simulink model "projectme548"  (R2016a)
settings: Solver=ode45  SolverMode=SingleTasking  StartTime=0.0  StopTime=5  MaxStep=0.01  RelTol=1e-3
model workspace (MAT data in the model file):
  A = 29.46
  Cd = 0.27
  Converter_K = [105 107 109 110 111 118 120 130 140 158 600]
  Converter_K2 = [138 139 138 138 139 140 142 145 155 165 200]
  Converter_K3 = [137.465208994; 137.065019157; 135.864449646; 135.664354728; 137.565256453; 140.366585312; 145.268910814; 152.872517717; 162.9773111; 164.27792807; 166.178829795; 167.979684062; 170.080680706; 172.781962105; 175.383196045; 179.585189333; 183.587087703; 189.890077635; 197.693779455; 215.902417037; 244.515990379]
  Converter_sratio = [0 0.1 0.2 0.3 0.4 0.5 0.6 0.7 0.8 0.9 1]
  Converter_sratio3 = [0 0.1 0.2 0.3 0.4 0.5 0.6 0.7 0.8 0.81 0.82 0.83 0.84 0.85 0.86 0.87 0.88 0.89 0.9 0.92 0.94]
  Converter_tratio = [2.1 2.03 1.93 1.82 1.7 1.58 1.42 1.3 1.17 1 1]
  Converter_tratio3 = [2.232 2.075 1.975 1.846 1.72 1.564 1.409 1.254 1.096 1.08 1.061 1.043 1.028 1.012 1.002 1.002 1.001 0.998 1 1.001 1.002]
  Engine_speed = [1000 1500 2000 2500 3000 3500 4000 4500 5000 5500 6000 6500 7000]
  Engine_torque = [140 152 156 167 164 167 169 175 171 165 159 150 138]
  Engine_torque2 = [160 170 185 190 198 205 210 170 160 150 140 145 120]
  Engine_torque3 = [134.973873267 156.363175588 165.213921376 168.901732121 173.327105015 175.539791462 173.327105015 169.63929427 162.26367278 147.5124298 132.76118682 88.50745788 59.00497192]
  G = 0
  I_c1r2 = 0.02
  I_c2r3 = 0.02
  I_input = 0.02
  I_out = 0.02
  I_s1 = 0.02
  I_s3 = 0.02
  Iv = 8.97221507589
  Je = 0.3
  T_C = [0 7 11.9677 49 80.1613 93.2581 98.6774 99.129 98.6774 98.2258 98.6774 99.5806 98.6774 98.2258 97.3226 102.2903 109.9677 133.4516 134.3548]
  W = 3472
  ans = 0.94
  f = 0.018
  g = 32.2
  ia = 2.6
  r = 0.75
undefined symbols (not defined in the file): magnitude, sigbuilder_block
settings Model: PauseTimes=1  Creator=eiddie  LastModifiedBy=xiaohuil
settings DataIOCC: LimitDataPoints=on  SaveFormat=Array
settings OptimizationCC: BlockReduction=off  BooleanDataType=off
settings DebuggingCC: SaveWithParameterizedLinksMsg=none  UnderspecifiedInitializationDetection=Classic  MergeDetectMultiDrivingBlocksExec=none  SignalResolutionControl=TryResolveAllWithWarning
settings HardwareCC: ProdBitPerPointer=32  ProdLargestAtomicFloat=None  ProdIntDivRoundTo=Undefined  ProdEndianess=Unspecified  ProdWordSize=32  ProdHWDeviceType=32-bit Generic  TargetUnknown=on
settings ModelReferenceCC: PropagateSignalLabelsOutOfModel=off
settings ConfigComp: CovModelRefEnable=Off  CovSFcnEnable=off

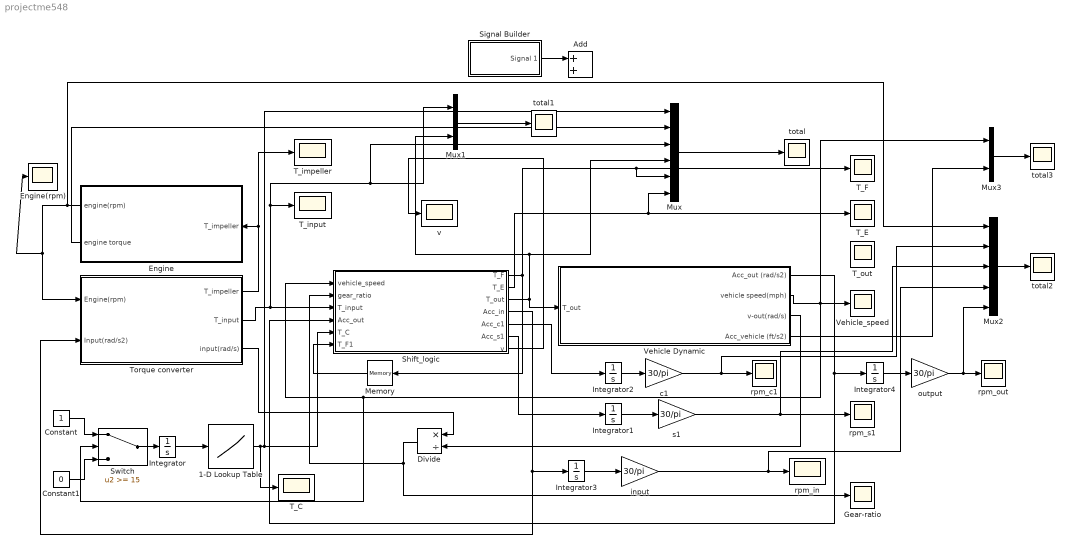
== system projectme548 ==
  1-D Lookup Table : Lookup_n-D  NumberOfTableDimensions=1  BreakpointsForDimension1=[0,0.1,0.2,0.3,0.4,0.5,0.6,0.7,0.8,0.9,1,1.1,1.2,1.3,1.4,1.5,1.6,1.7,1.8]  Table=T_C  InternalRulePriority=Speed  RndMeth=Simplest  InputSameDT=on
  Add : Sum
  Constant : Constant
  Constant1 : Constant  Value=0
  Divide : Product  Inputs=*/
  Engine : Subsystem
  Engine(rpm) : Scope
  Gear-ratio : Scope
  Integrator{,1..4} (5 alike) : Integrator
  Memory : Memory  X0=1
  Mux : Mux  Inputs=6
  Mux1 : Mux  Inputs=2
  Mux2 : Mux  Inputs=5
  Mux3 : Mux  Inputs=2
  Shift_logic : MATLAB Function  TreatAsAtomicUnit=on
      settings: MinAlgLoopOccurrences=on
  Signal Builder : Subsystem  Tag=STV Subsys  LoadFcn=sigbuilder_block('load');  StartFcn=sigbuilder_block('start');  StopFcn=sigbuilder_block('stop');  ClipboardFcn=sigbuilder_block('clipboard');  mask(Sigbuilder block){}
      mask help: Simulink:masks:SigbuilderBlock_MD
      mask init:
      | if ~strcmp(get_param(bdroot(gcbh),'SimulationStatus'),'stopped') tuvar = sigbuilder_block('maskInit'); end
      settings: CopyFcn=sigbuilder_block('copy');  DeleteFcn=sigbuilder_block('delete');  ModelCloseFcn=sigbuilder_block('modelClose');  PreSaveFcn=sigbuilder_block('preSave');  PauseFcn=sigbuilder_block('pause');  ContinueFcn=sigbuilder_block('continue');  NameChangeFcn=sigbuilder_block('namechange');  OpenFcn=sigbuilder_block('open',[437.6 199.2 550.4 400 ]);  CloseFcn=sigbuilder_block('close');
      mask Display: plot(0, 0, 100, 100,[2, 2, 32, 32, 2], [68, 8, 8, 68, 68],[32, 2], [38, 38], [32, 19, 2],[53, 60, 44], [32, 17, 17, 2],[16, 16, 31, 31]);txt = getActiveGroup(gcbh);text(2, 100, txt,'verticalAlignment', 'top');
  Switch : Switch  Threshold=15
  T_C : Scope
  T_E : Scope
  T_F : Scope
  T_impeller : Scope
  T_input : Scope
  T_out : Scope
  Torque converter : Subsystem
  Vehicle Dynamic : Subsystem
  Vehicle_speed : Scope
  c1 : Gain  Gain=30/pi
  input : Gain  Gain=30/pi
  output : Gain  Gain=30/pi
  rpm_c1 : Scope
  rpm_in : Scope
  rpm_out : Scope
  rpm_s1 : Scope
  s1 : Gain  Gain=30/pi
  total{,1..3} (4 alike) : Scope
  "v " : Scope
  wires:
  Engine/1(engine(rpm)) -> Torque converter/1(Engine(rpm)), Engine(rpm)/1, Mux2/1
  Torque converter/1(T_impeller) -> T_impeller/1, Engine/1(T_impeller)
  Torque converter/2(T_input) -> Shift_logic/3(T_input), Mux1/1, Mux/3, T_input/1
  Shift_logic/3(T_out) -> Mux1/2, Mux/4, Vehicle Dynamic/1(T_out)
  Shift_logic/2(T_E) -> Mux/6, T_E/1
  Shift_logic/6(Acc_s1) -> Integrator1/1
  Constant1/1 -> Switch/3
  Constant/1 -> Switch/1
  Switch/1 -> Integrator/1
  Integrator/1 -> 1-D Lookup Table/1
  1-D Lookup Table/1 -> Mux/1, Shift_logic/5(T_C), T_C/1
  Shift_logic/1(T_F) -> Memory/1, Mux/5, T_F/1
  Vehicle Dynamic/3(v-out(rad/s)) -> Divide/2
  Torque converter/3(input(rad/s)) -> Divide/1
  Memory/1 -> Shift_logic/6(T_F1)
  Shift_logic/7(v) -> "v "/1
  Vehicle Dynamic/2(vehicle speed(mph)) -> Mux3/1, Switch/2, Shift_logic/1(vehicle_speed), Vehicle_speed/1
  Vehicle Dynamic/1(Acc_out (rad/s2)) -> Shift_logic/4(Acc_out), Integrator4/1
  Shift_logic/4(Acc_in) -> Integrator3/1, Torque converter/2(Input(rad/s2))
  Divide/1 -> Shift_logic/2(gear_ratio), Gear-ratio/1
  Mux/1 -> total/1
  Engine/2(engine torque) -> Mux/2
  Mux1/1 -> total1/1
  Integrator1/1 -> s1/1
  Shift_logic/5(Acc_c1) -> Integrator2/1
  Integrator2/1 -> c1/1
  s1/1 -> Mux2/3, rpm_s1/1
  c1/1 -> Mux2/2, rpm_c1/1
  Integrator3/1 -> input/1
  input/1 -> Mux2/4, rpm_in/1
  Integrator4/1 -> output/1
  output/1 -> Mux2/5, rpm_out/1
  Mux2/1 -> total2/1
  Vehicle Dynamic/4(Acc_vehicle (ft/s2)) -> Mux3/2
  Mux3/1 -> total3/1
  Signal Builder/1(Signal 1) -> Add/1

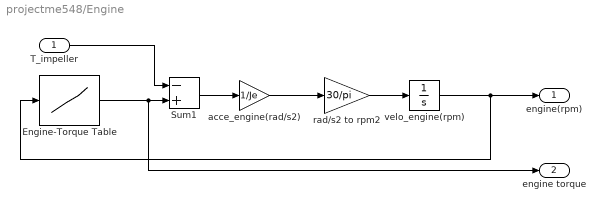
== system projectme548/Engine ==
  T_impeller : Inport
  Engine-Torque Table : Lookup_n-D  NumberOfTableDimensions=1  BreakpointsForDimension1=Engine_speed  Table=Engine_torque3  InternalRulePriority=Speed  RndMeth=Simplest  InputSameDT=on
  Sum1 : Sum  Inputs=-+  SaturateOnIntegerOverflow=on  InputSameDT=on  OutDataTypeStr=Inherit: Same as first input
  acce_engine(rad/s2) : Gain  Gain=1/Je
  rad/s2 to rpm2 : Gain  Gain=30/pi
  velo_engine(rpm) : Integrator  InitialCondition=1000  UpperSaturationLimit=7000  LowerSaturationLimit=700
  engine(rpm) : Outport
  engine torque : Outport  Port=2
  wires:
  Engine-Torque Table/1 -> engine torque/1, Sum1/2
  Sum1/1 -> acce_engine(rad/s2)/1
  T_impeller/1 -> Sum1/1
  acce_engine(rad/s2)/1 -> rad/s2 to rpm2/1
  rad/s2 to rpm2/1 -> velo_engine(rpm)/1
  velo_engine(rpm)/1 -> Engine-Torque Table/1, engine(rpm)/1

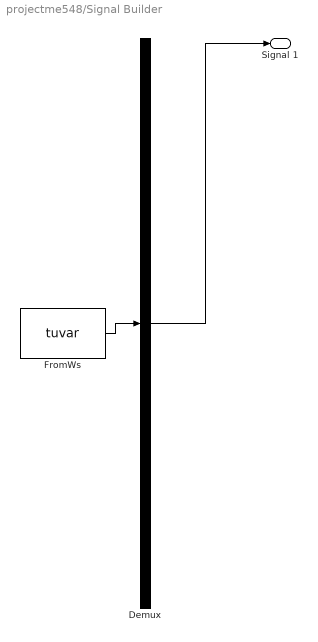
== system projectme548/Signal Builder ==
  Demux : Demux  Tag=STV Demux  Outputs=1
  FromWs : FromWorkspace  Tag=STV FromWs  VariableName=tuvar  SampleTime=0
      SigBuilderData=|
      | common.afterFinalStr = 'Extrapolate'
      | common.sampleTime = 0
      | dataSet.timeRange = [0 10]
      | dataSet.name = 'Group 1'
      | sbobj.Groups.Name = 'Group 1'
      | sbobj.Groups.Signals.Name = 'Signal 1'
      | sbobj.Groups.Signals.XData = [0 1.7 1.77 1.85 6 10]
      | sbobj.Groups.Signals.YData = [0 0 100 0 0 0]
  Signal 1 : Outport  Tag=STV Outport
  wires:
  Demux/1 -> Signal 1/1
  FromWs/1 -> Demux/1

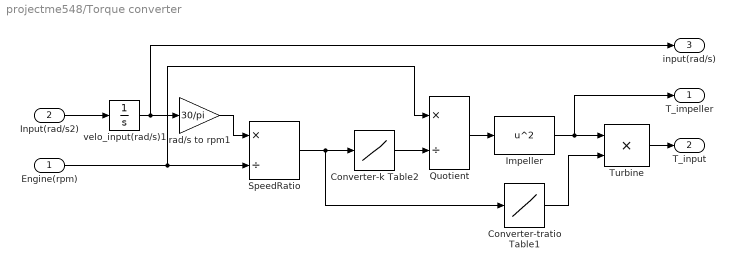
== system projectme548/Torque converter ==
  Engine(rpm) : Inport
  Input(rad/s2) : Inport  Port=2
  Converter-k Table2 : Lookup_n-D  NumberOfTableDimensions=1  BreakpointsForDimension1=Converter_sratio  Table=Converter_K  InternalRulePriority=Speed  RndMeth=Simplest  InputSameDT=on
  Converter-tratio Table1 : Lookup_n-D  NumberOfTableDimensions=1  BreakpointsForDimension1=Converter_sratio  Table=Converter_tratio  InternalRulePriority=Speed  RndMeth=Simplest  InputSameDT=on
  Impeller : Fcn  Expr=u^2
  Quotient : Product  Inputs=*/  SaturateOnIntegerOverflow=on  InputSameDT=on  OutDataTypeStr=Inherit: Same as first input
  SpeedRatio : Product  Inputs=*/  SaturateOnIntegerOverflow=on  InputSameDT=on  OutDataTypeStr=Inherit: Same as first input
  Turbine : Product  SaturateOnIntegerOverflow=on  InputSameDT=on  OutDataTypeStr=Inherit: Same as first input
  rad/s to rpm1 : Gain  Gain=30/pi
  velo_input(rad/s)1 : Integrator
  T_impeller : Outport
  T_input : Outport  Port=2
  input(rad/s) : Outport  Port=3
  wires:
  Converter-tratio Table1/1 -> Turbine/2
  Quotient/1 -> Impeller/1
  Converter-k Table2/1 -> Quotient/2
  Impeller/1 -> T_impeller/1, Turbine/1
  Turbine/1 -> T_input/1
  Engine(rpm)/1 -> SpeedRatio/2, Quotient/1
  rad/s to rpm1/1 -> SpeedRatio/1
  velo_input(rad/s)1/1 -> input(rad/s)/1, rad/s to rpm1/1
  Input(rad/s2)/1 -> velo_input(rad/s)1/1
  SpeedRatio/1 -> Converter-tratio Table1/1, Converter-k Table2/1

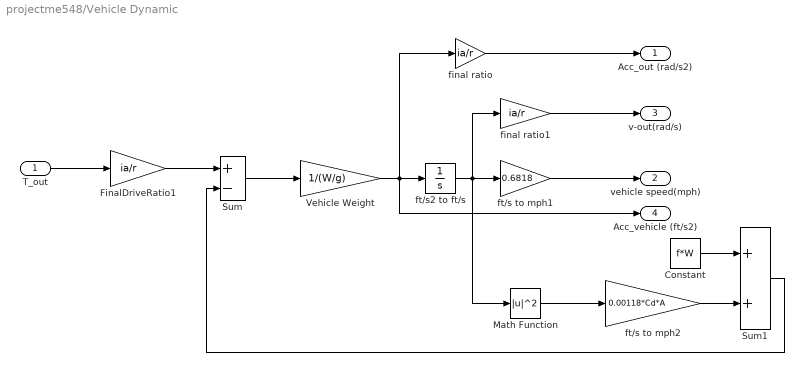
== system projectme548/Vehicle Dynamic ==
  T_out : Inport
  Constant : Constant  Value=f*W
  FinalDriveRatio1 : Gain  Gain=ia/r  SaturateOnIntegerOverflow=on  OutDataTypeStr=Inherit: Same as input  ParamDataTypeStr=Inherit: Same as input
  Math Function : Math  Operator=magnitude^2  SaturateOnIntegerOverflow=on
  Sum : Sum  Inputs=+-  SaturateOnIntegerOverflow=on  InputSameDT=on  OutDataTypeStr=Inherit: Same as first input
  Sum1 : Sum  SaturateOnIntegerOverflow=on  InputSameDT=on  OutDataTypeStr=Inherit: Same as first input
  Vehicle Weight : Gain  Gain=1/(W/g)  SaturateOnIntegerOverflow=on  OutDataTypeStr=Inherit: Same as input  ParamDataTypeStr=Inherit: Same as input
  final ratio : Gain  Gain=ia/r
  final ratio1 : Gain  Gain=ia/r
  ft/s to mph1 : Gain  Gain=0.6818
  ft/s to mph2 : Gain  Gain=0.00118*Cd*A
  ft/s2 to ft/s : Integrator
  Acc_out (rad/s2) : Outport
  vehicle speed(mph) : Outport  Port=2
  v-out(rad/s) : Outport  Port=3
  Acc_vehicle (ft/s2) : Outport  Port=4
  wires:
  T_out/1 -> FinalDriveRatio1/1
  FinalDriveRatio1/1 -> Sum/1
  Sum/1 -> Vehicle Weight/1
  Vehicle Weight/1 -> Acc_vehicle (ft/s2)/1, final ratio/1, ft/s2 to ft/s/1
  ft/s2 to ft/s/1 -> Math Function/1, final ratio1/1, ft/s to mph1/1
  ft/s to mph1/1 -> vehicle speed(mph)/1
  Math Function/1 -> ft/s to mph2/1
  Constant/1 -> Sum1/1
  ft/s to mph2/1 -> Sum1/2
  Sum1/1 -> Sum/2
  final ratio/1 -> Acc_out (rad/s2)/1
  final ratio1/1 -> v-out(rad/s)/1

== matlab function projectme548/Shift_logic ==
  data: vehicle_speed input; T_F output; gear_ratio input; T_input input; Acc_out input; T_C input; T_E output; T_out output; Acc_in output; Acc_c1 output; Acc_s1 output; T_F1 input; v output
function [T_F,T_E,T_out,Acc_in,Acc_c1,Acc_s1,v] = fcn(vehicle_speed,gear_ratio,T_input,Acc_out,T_C,T_F1)
i1=1/0.223;
i2=2.8722;
I_input=0.02;
I_c2r3=0.02;
I_s1=0.02;
I_s3=0.02;
I_c1r2=0.02;
I_out=0.02;
T_F=0;
T_E=0;
T_out=0;
Acc_in=0;
Acc_c1=0;
Acc_s1=0;
v=0;
if (vehicle_speed<15)
    Acc_in=Acc_out/0.223;
    T_out=4.4837*T_input-4.4837*I_input*Acc_in-0.4459*I_c2r3*Acc_in-1.8528*I_s1*Acc_in-0.223*I_out*Acc_in;
    T_F=2.1707*T_input-2.1707*I_input*Acc_in-2.4956*I_s1*Acc_in;
    T_E=1.3131*T_input-1.3131*I_input*Acc_in-0.1306*I_c2r3*Acc_in;
    Acc_s1=-0.6428*Acc_in;
    Acc_c1=0;
else if (vehicle_speed>=15&&T_F1>0)
        Acc_in=Acc_out/0.223;
        T_out=4.4837*T_input-4.4837*I_input*Acc_in-0.4459*I_c2r3*Acc_in-2.8824*T_C-1.8528*I_s1*Acc_in-0.223*I_out*Acc_in;
        T_F=2.1707*T_input-2.1707*I_input*Acc_in-2.4956*I_s1*Acc_in-3.8824*T_C;
        T_E=1.3131*T_input-1.3131*I_input*Acc_in-0.1306*I_c2r3*Acc_in;
        Acc_s1=-0.6428*Acc_in;
        Acc_c1=0;
        v=3;
    else if (vehicle_speed>15&&gear_ratio>i2&&T_F1<=0)
            a=0.8*T_input;
            Acc_in=(Acc_out*(2.0656*I_c1r2+19.9443*I_s1)-3.8824*T_C+2.1707*a)/(0.4607*I_c1r2+6.9441*I_s1+2.1707*I_input);
            T_out=4.4838*a-4.4838*I_input*Acc_in-1.9997*I_c2r3*Acc_out-2.8824*T_C+14.8072*I_s1*Acc_out-5.1555*I_s1*Acc_in-I_out*Acc_out;
            T_E=1.3131*a-1.3131*I_input*Acc_in-0.5856*I_c2r3*Acc_out;
            Acc_c1=2.0656*Acc_out-0.4607*Acc_in;
            Acc_s1=5.1371*Acc_out-1.7886*Acc_in;
            T_F=0;
            v=2;
        else if(vehicle_speed>15&&gear_ratio<=i2)
            Acc_in=2.8722*Acc_out;
            c=0.5591*T_input-1.6059*I_input*Acc_out+0.1912*I_c1r2*Acc_out;
            T_E=1.3131*T_input-3.7716*I_input*Acc_out+0.5856*I_c2r3*Acc_out;
            T_out=3.4146*T_E-2.8824*c-I_out*Acc_out;
            Acc_c1=0.7424*Acc_out;
            Acc_c2=1.4141*Acc_out;
            Acc_s1=0;
            T_F=0;
            v=0;
        end
end

end
end
